simulink model "pendsimples"  (R2022a)
settings: Solver=VariableStepAuto  StartTime=0.0  StopTime=100  RelTol=1e-6
settings Model: Creator=PC  LastModifiedBy=PC

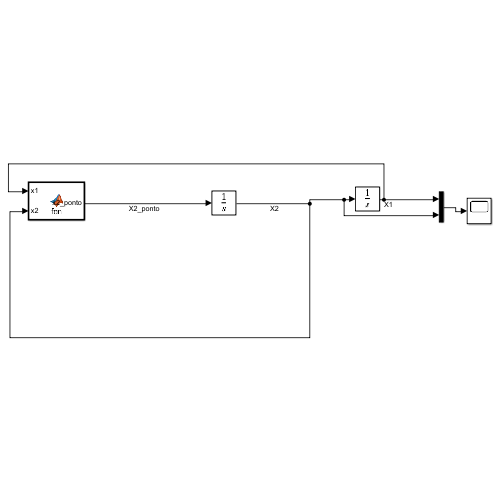
[thumbnail: Simulink's stored preview of the top-level diagram]
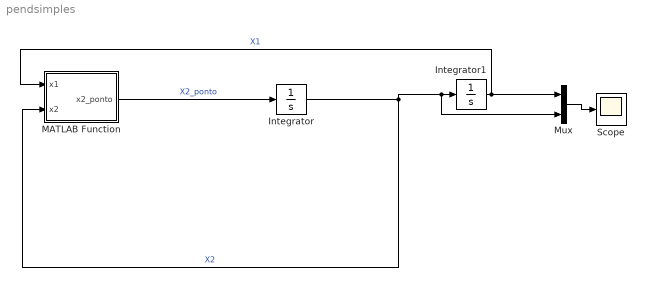
== system pendsimples ==
  Integrator : Integrator
  Integrator1 : Integrator  InitialCondition=pi/2
  MATLAB Function : MATLAB Function  TreatAsAtomicUnit=on
  Mux : Mux  Inputs=2
  Scope : Scope
  wires:
  Integrator/1 -> Mux/2, Integrator1/1, MATLAB Function/2(x2)  "X2"
  MATLAB Function/1(x2_ponto) -> Integrator/1  "X2_ponto"
  Integrator1/1 -> MATLAB Function/1(x1), Mux/1  "X1"
  Mux/1 -> Scope/1

== matlab function pendsimples/MATLAB Function ==
  data: x1 input; x2_ponto output; x2 input
function x2_ponto = fcn(x1,x2)

a=1;b=0;
x2_ponto=-a*sin(x1)-b*x2;
